simulink model "autopilot_simulink"  (R2016a)
settings: Solver=ode3  StartTime=0.0  StopTime=20  FixedStep=0.01  RelTol=1e-3
values from neighbouring files (symbols this model uses):
  Kx = KK(:,1:8)    [drone_config.m]
  Ky = KK(:,9:12)    [drone_config.m]
undefined symbols (not defined in the file or in its folder): sigbuilder_block
libraries: aerolibtransform2 x1, aerolib6dof2 x1
settings Model: Creator=rcasado  LastModifiedBy=rcasado
settings DataIOCC: LimitDataPoints=on  SaveFormat=Array
settings DebuggingCC: MultiTaskRateTransMsg=warning  AllowSymbolicDim=off
settings HardwareCC: ProdBitPerPointer=32  ProdLargestAtomicFloat=None  ProdIntDivRoundTo=Undefined  ProdEndianess=Unspecified  ProdWordSize=32  ProdHWDeviceType=32-bit Generic
settings ModelReferenceCC: PropagateSignalLabelsOutOfModel=off
settings ConfigComp: CovModelRefEnable=Off

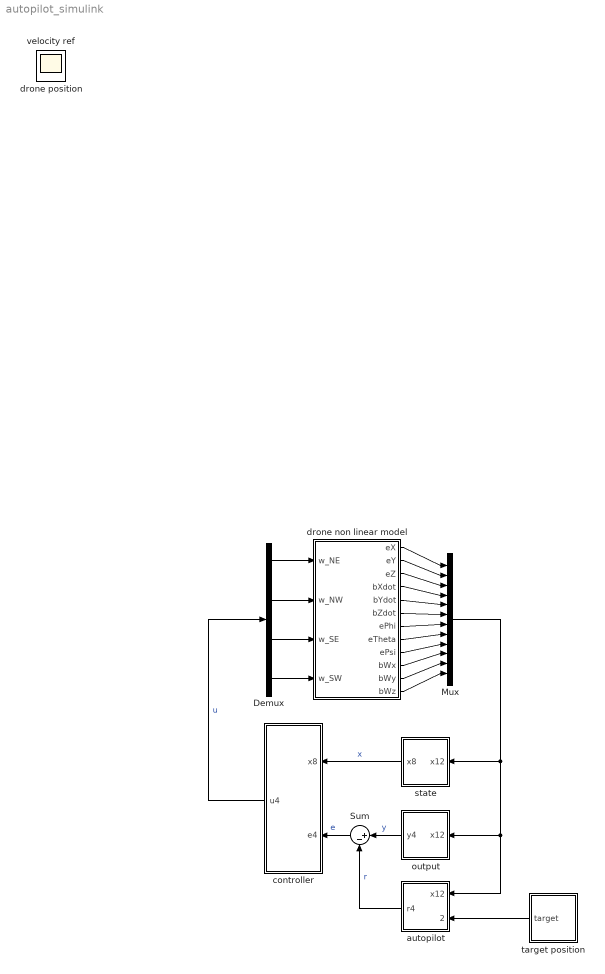
== system autopilot_simulink ==
  Demux : Demux
  Mux : Mux  Inputs=12
  Sum : Sum  Inputs=|+-
  autopilot : Subsystem
  controller : Subsystem
  drone non linear model : Subsystem
  output : Subsystem
  state : Subsystem
  target position : Subsystem
  drone position : Scope
  velocity ref : Scope
  wires:
  Mux/1 -> autopilot/1(x12), output/1(x12), state/1(x12)
  autopilot/1(r4) -> Sum/2  "r"
  output/1(y4) -> Sum/1  "y"
  state/1(x8) -> controller/1(x8)  "x"
  Sum/1 -> controller/2(e4)  "e"
  drone non linear model/1(eX) -> Mux/1
  drone non linear model/3(eZ) -> Mux/3
  drone non linear model/2(eY) -> Mux/2
  Demux/1 -> drone non linear model/1(w_NE)
  Demux/2 -> drone non linear model/2(w_NW)
  Demux/3 -> drone non linear model/3(w_SE)
  Demux/4 -> drone non linear model/4(w_SW)
  drone non linear model/12(bWz) -> Mux/12
  drone non linear model/11(bWy) -> Mux/11
  drone non linear model/4(bXdot) -> Mux/4
  drone non linear model/5(bYdot) -> Mux/5
  drone non linear model/6(bZdot) -> Mux/6
  drone non linear model/7(ePhi) -> Mux/7
  drone non linear model/8(eTheta) -> Mux/8
  drone non linear model/9(ePsi) -> Mux/9
  drone non linear model/10(bWx) -> Mux/10
  controller/1(u4) -> Demux/1  "u"
  target position/1(target) -> autopilot/2(target)

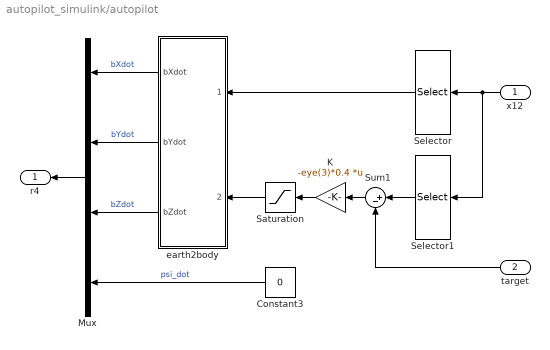
== system autopilot_simulink/autopilot ==
  x12 : Inport
  target : Inport  Port=2
  Constant3 : Constant  Value=0
  K : Gain  Gain=-eye(3)*0.4  Multiplication=Matrix(K*u)
  Mux : Mux
  Saturation : Saturate  UpperLimit=2  LowerLimit=-2
  Selector : Selector  InputPortWidth=12  IndexOptions=Index vector (dialog)  Indices=[7,8,9]  OutputSizes=1
  Selector1 : Selector  InputPortWidth=12  IndexOptions=Index vector (dialog)  Indices=[1;2;3]  OutputSizes=1
  Sum1 : Sum  Inputs=|+-
  earth2body : Subsystem
  r4 : Outport
  wires:
  Mux/1 -> r4/1
  Saturation/1 -> earth2body/2(eXYZdot)
  Constant3/1 -> Mux/4  "psi_dot"
  earth2body/2(bYdot) -> Mux/2  "bYdot"
  earth2body/1(bXdot) -> Mux/1  "bXdot"
  earth2body/3(bZdot) -> Mux/3  "bZdot"
  Selector1/1 -> Sum1/1
  K/1 -> Saturation/1
  Sum1/1 -> K/1
  x12/1 -> Selector1/1, Selector/1
  target/1 -> Sum1/2
  Selector/1 -> earth2body/1(orientation)

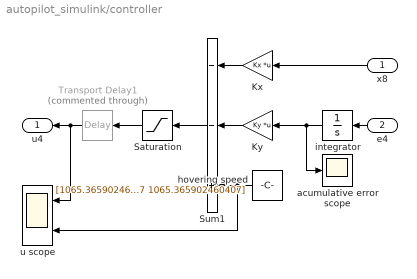
== system autopilot_simulink/controller ==
  x8 : Inport
  e4 : Inport  Port=2
  Kx : Gain  Gain=Kx  Multiplication=Matrix(K*u)
  Ky : Gain  Gain=Ky  Multiplication=Matrix(K*u)
  Saturation : Saturate  UpperLimit=1650  LowerLimit=0
  Sum1 : Sum  Inputs=--+
  Transport Delay1 : TransportDelay  Commented=through  DelayTime=0.05
  acumulative error scope : Scope
  hovering speed : Constant  Value=[1065.365902460407 1065.365902460407 1065.365902460407 1065.365902460407]
  integrator : Integrator
  u scope : Scope  NumInputPorts=2
  u4 : Outport
  wires:
  Saturation/1 -> Transport Delay1/1
  Kx/1 -> Sum1/1
  x8/1 -> Kx/1
  hovering speed/1 -> u scope/2, Sum1/3
  Sum1/1 -> Saturation/1
  Transport Delay1/1 -> u scope/1, u4/1
  e4/1 -> integrator/1
  Ky/1 -> Sum1/2
  integrator/1 -> Ky/1, acumulative error scope/1

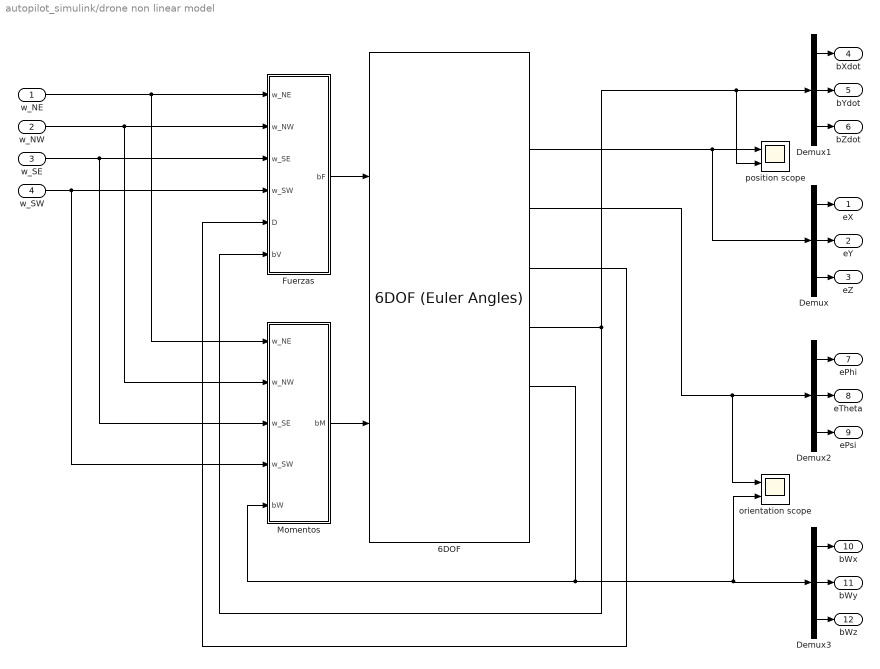
== system autopilot_simulink/drone non linear model ==
  w_NE : Inport
  w_NW : Inport  Port=2
  w_SE : Inport  Port=3
  w_SW : Inport  Port=4
  6DOF : aerolib6dof2/6DOF (Euler Angles)  units=Metric (MKS)  mtype=Fixed  rep=Euler Angles  xme_0=[0 0 10]  Vm_0=[0 0 0]  eul_0=[0 0 deg2rad(-30)]  pm_0=[0 0 0]  mass_0=1.840  mass_e=0.5  mass_f=2.0  inertia="[0.024916667  0  0 ; 0 0.024916667 0 ; 0 0 0.049066667]"  inertia_e=eye(3)  inertia_f=2*eye(3)  k_quat=1.0  vre_flag=on
  Demux{,1..3} (4 alike) : Demux  Outputs=3
  Fuerzas : Subsystem
  Momentos : Subsystem
  orientation scope : Scope  NumInputPorts=2
  position scope : Scope  NumInputPorts=2
  eX : Outport
  eY : Outport  Port=2
  eZ : Outport  Port=3
  bXdot : Outport  Port=4
  bYdot : Outport  Port=5
  bZdot : Outport  Port=6
  ePhi : Outport  Port=7
  eTheta : Outport  Port=8
  ePsi : Outport  Port=9
  bWx : Outport  Port=10
  bWy : Outport  Port=11
  bWz : Outport  Port=12
  wires:
  6DOF/2 -> Demux/1, position scope/1
  Momentos/1(bM) -> 6DOF/2
  w_NE/1 -> Momentos/1(w_NE), Fuerzas/1(w_NE)
  w_NW/1 -> Momentos/2(w_NW), Fuerzas/2(w_NW)
  w_SE/1 -> Momentos/3(w_SE), Fuerzas/3(w_SE)
  w_SW/1 -> Momentos/4(w_SW), Fuerzas/4(w_SW)
  6DOF/4 -> Fuerzas/5(D)
  Fuerzas/1(bF) -> 6DOF/1
  6DOF/6 -> Demux3/1, orientation scope/2, Momentos/5(bW)
  Demux/1 -> eX/1
  Demux/2 -> eY/1
  Demux/3 -> eZ/1
  6DOF/5 -> position scope/2, Demux1/1, Fuerzas/6(bV)
  Demux1/1 -> bXdot/1
  Demux1/2 -> bYdot/1
  Demux1/3 -> bZdot/1
  Demux2/1 -> ePhi/1
  Demux2/2 -> eTheta/1
  Demux2/3 -> ePsi/1
  Demux3/1 -> bWx/1
  Demux3/2 -> bWy/1
  Demux3/3 -> bWz/1
  6DOF/3 -> orientation scope/1, Demux2/1

== system autopilot_simulink/output ==
  x12 : Inport
  Selector : Selector  InputPortWidth=12  IndexOptions=Index vector (dialog)  Indices=[4 5 6 12]  OutputSizes=1
  y4 : Outport
  wires:
  x12/1 -> Selector/1
  Selector/1 -> y4/1

== system autopilot_simulink/state ==
  x12 : Inport
  Selector : Selector  InputPortWidth=12  IndexOptions=Index vector (dialog)  Indices=[7 8 10 11 12 4 5 6]  OutputSizes=1
  x8 : Outport
  wires:
  x12/1 -> Selector/1
  Selector/1 -> x8/1

== system autopilot_simulink/target position ==
  Mux1 : Mux  Inputs=3
  target position : Subsystem  Tag=STV Subsys  LoadFcn=sigbuilder_block('load',[514.2 0.6 340.2 585.6 ]);  StartFcn=sigbuilder_block('start');  StopFcn=sigbuilder_block('stop');  ClipboardFcn=sigbuilder_block('clipboard');  mask(Sigbuilder block){}
      mask help: Simulink:masks:SigbuilderBlock_MD
      mask init:
      | if ~strcmp(get_param(bdroot(gcbh),'SimulationStatus'),'stopped') tuvar = sigbuilder_block('maskInit'); end
      settings: CopyFcn=sigbuilder_block('copy');  DeleteFcn=sigbuilder_block('delete');  ModelCloseFcn=sigbuilder_block('modelClose');  PreSaveFcn=sigbuilder_block('preSave');  PauseFcn=sigbuilder_block('pause');  ContinueFcn=sigbuilder_block('continue');  NameChangeFcn=sigbuilder_block('namechange');  OpenFcn=sigbuilder_block('open',[514.2 0.6 375 585.6 ]);  CloseFcn=sigbuilder_block('close');
      mask Display: plot(0, 0, 100, 100,[2, 2, 32, 32, 2], [68, 8, 8, 68, 68],[32, 2], [38, 38], [32, 19, 2],[53, 60, 44], [32, 17, 17, 2],[16, 16, 31, 31]);txt = getActiveGroup(gcbh);text(2, 100, txt,'verticalAlignment', 'top');
  target : Outport
  wires:
  target position/3(pos_z) -> Mux1/3
  target position/1(pos_x) -> Mux1/1
  target position/2(pos_y) -> Mux1/2
  Mux1/1 -> target/1

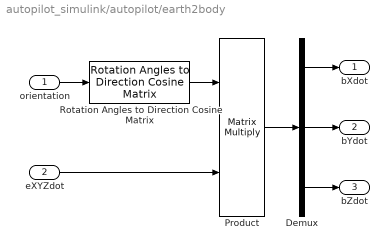
== system autopilot_simulink/autopilot/earth2body ==
  orientation : Inport
  eXYZdot : Inport  Port=2
  Demux : Demux  Outputs=3
  Product : Product  Multiplication=Matrix(*)
  Rotation Angles to Direction Cosine Matrix : aerolibtransform2/Rotation Angles to Direction Cosine Matrix  rotationOrder=XYZ
  bXdot : Outport
  bYdot : Outport  Port=2
  bZdot : Outport  Port=3
  wires:
  Product/1 -> Demux/1
  Rotation Angles to Direction Cosine Matrix/1 -> Product/1
  eXYZdot/1 -> Product/2
  orientation/1 -> Rotation Angles to Direction Cosine Matrix/1
  Demux/1 -> bXdot/1
  Demux/2 -> bYdot/1
  Demux/3 -> bZdot/1

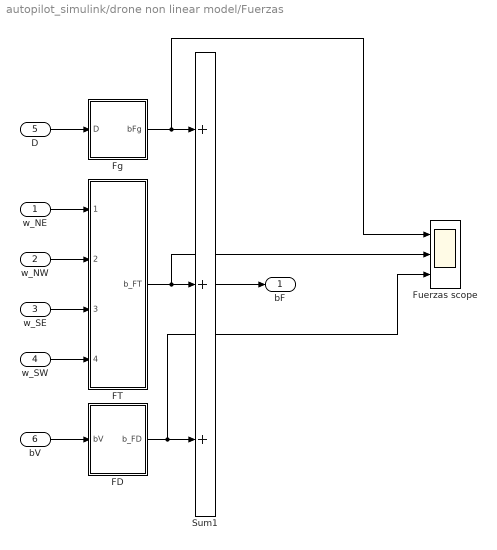
== system autopilot_simulink/drone non linear model/Fuerzas ==
  w_NE : Inport
  w_NW : Inport  Port=2
  w_SE : Inport  Port=3
  w_SW : Inport  Port=4
  D : Inport  Port=5
  bV : Inport  Port=6
  FD : Subsystem
  FT : Subsystem
  Fg : Subsystem
  Fuerzas scope : Scope  NumInputPorts=3
  Sum1 : Sum  Inputs=+++
  bF : Outport
  wires:
  D/1 -> Fg/1(D)
  Fg/1(bFg) -> Fuerzas scope/1, Sum1/1
  FT/1(b_FT) -> Fuerzas scope/2, Sum1/2
  w_SW/1 -> FT/4(w_SW)
  w_NE/1 -> FT/1(w_NE)
  w_SE/1 -> FT/3(w_SE)
  w_NW/1 -> FT/2(w_NW)
  Sum1/1 -> bF/1
  bV/1 -> FD/1(bV)
  FD/1(b_FD) -> Sum1/3, Fuerzas scope/3

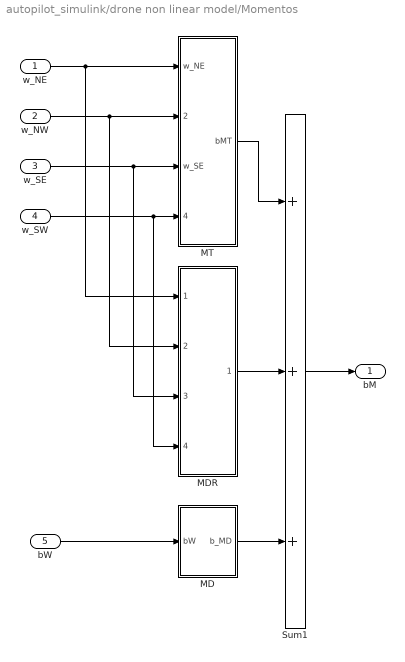
== system autopilot_simulink/drone non linear model/Momentos ==
  w_NE : Inport
  w_NW : Inport  Port=2
  w_SE : Inport  Port=3
  w_SW : Inport  Port=4
  bW : Inport  Port=5
  MD : Subsystem
  MDR : Subsystem
  MT : Subsystem
  Sum1 : Sum  Inputs=+++
  bM : Outport
  wires:
  bW/1 -> MD/1(bW)
  MT/1(bMT) -> Sum1/1
  w_SW/1 -> MDR/4(w_SW), MT/4(w_SW)
  w_NE/1 -> MDR/1(w_NE), MT/1(w_NE)
  w_SE/1 -> MDR/3(w_SE), MT/3(w_SE)
  w_NW/1 -> MDR/2(w_NW), MT/2(w_NW)
  Sum1/1 -> bM/1
  MD/1(b_MD) -> Sum1/3
  MDR/1(b_MDR) -> Sum1/2

== system autopilot_simulink/target position/target position ==
  Demux : Demux  Tag=STV Demux  Outputs=3
  FromWs : FromWorkspace  Tag=STV FromWs  VariableName=tuvar  SampleTime=0
      SigBuilderData=|
      | common.afterFinalStr = 'Extrapolate'
      | common.sampleTime = 0
      | dataSet(1).timeRange = [0 20]
      | dataSet(1).name = 've y aterriza'
      | dataSet(2).timeRange = [0 10]
      | dataSet(2).name = 'avanza1'
      | sbobj.Groups(1).Name = 've y aterriza'
      | sbobj.Groups(1).Signals(1).Name = 'pos_x'
      | sbobj.Groups(1).Signals(1).XData = [0 20]
      | sbobj.Groups(1).Signals(1).YData = [4 4]
      | sbobj.Groups(1).Signals(2).Name = 'pos_y'
      | sbobj.Groups(1).Signals(2).XData = [0 5 20]
      | sbobj.Groups(1).Signals(2).YData = [0 4 4]
      | sbobj.Groups(1).Signals(3).Name = 'pos_z'
      | sbobj.Groups(1).Signals(3).XData = [0 5 15 20]
      | sbobj.Groups(1).Signals(3).YData = [10 10 0 0]
      | sbobj.Groups(1).TimeRange = [0 20]
      | sbobj.Groups(2).Name = 'avanza1'
      | sbobj.Groups(2).Signals(1).Name = 'pos_x'
      | sbobj.Groups(2).Signals(1).XData = [0 1 1 4 6 10]
      | sbobj.Groups(2).Signals(1).YData = [0 0 3 3 3 3]
      | sbobj.Groups(2).Signals(2).Name = 'pos_y'
      | sbobj.Groups(2).Signals(2).XData = [0 4 10]
      | sbobj.Groups(2).Signals(2).YData = [0 4 4]
      | sbobj.Groups(2).Signals(3).Name = 'pos_z'
      | sbobj.Groups(2).Signals(3).XData = [0 6 6 10]
      | sbobj.Groups(2).Signals(3).YData = [10 10 0 0]
  pos_x : Outport  Tag=STV Outport
  pos_y : Outport  Tag=STV Outport  Port=2
  pos_z : Outport  Tag=STV Outport  Port=3
  wires:
  FromWs/1 -> Demux/1
  Demux/1 -> pos_x/1
  Demux/2 -> pos_y/1
  Demux/3 -> pos_z/1

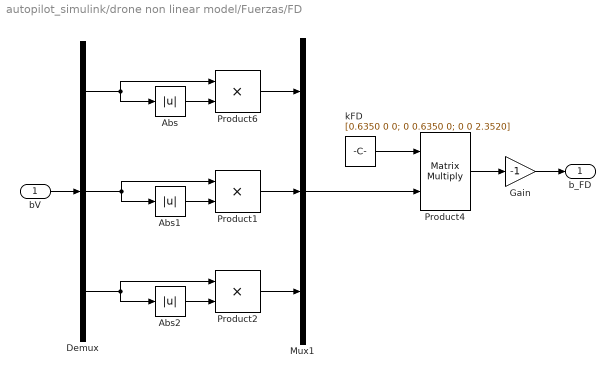
== system autopilot_simulink/drone non linear model/Fuerzas/FD ==
  bV : Inport
  Abs : Abs
  Abs1 : Abs
  Abs2 : Abs
  Demux : Demux  Outputs=3
  Gain : Gain  Gain=-1
  Mux1 : Mux  Inputs=3
  Product1 : Product
  Product2 : Product
  Product4 : Product  Multiplication=Matrix(*)
  Product6 : Product
  kFD : Constant  Value=[0.6350 0 0; 0 0.6350 0; 0 0 2.3520]
  b_FD : Outport
  wires:
  kFD/1 -> Product4/1
  Product4/1 -> Gain/1
  Mux1/1 -> Product4/2
  Product1/1 -> Mux1/2
  bV/1 -> Demux/1
  Abs/1 -> Product6/2
  Abs1/1 -> Product1/2
  Abs2/1 -> Product2/2
  Demux/1 -> Product6/1, Abs/1
  Demux/2 -> Product1/1, Abs1/1
  Demux/3 -> Product2/1, Abs2/1
  Product6/1 -> Mux1/1
  Product2/1 -> Mux1/3
  Gain/1 -> b_FD/1

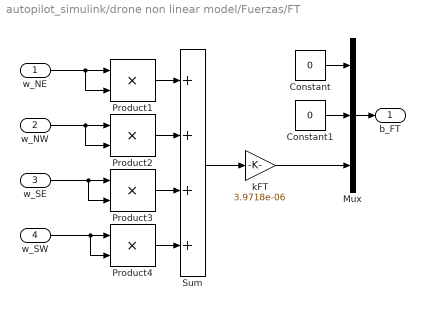
== system autopilot_simulink/drone non linear model/Fuerzas/FT ==
  w_NE : Inport
  w_NW : Inport  Port=2
  w_SE : Inport  Port=3
  w_SW : Inport  Port=4
  Constant : Constant  Value=0
  Constant1 : Constant  Value=0
  Mux : Mux  Inputs=3
  Product{1..4} (4 alike) : Product
  Sum : Sum  Inputs=++++
  kFT : Gain  Gain=3.9718e-06
  b_FT : Outport
  wires:
  Product4/1 -> Sum/4
  Product3/1 -> Sum/3
  Product2/1 -> Sum/2
  w_NW/1 -> Product2/2, Product2/1
  w_NE/1 -> Product1/2, Product1/1
  Product1/1 -> Sum/1
  Mux/1 -> b_FT/1
  w_SE/1 -> Product3/2, Product3/1
  w_SW/1 -> Product4/2, Product4/1
  Sum/1 -> kFT/1
  Constant/1 -> Mux/1
  Constant1/1 -> Mux/2
  kFT/1 -> Mux/3

== system autopilot_simulink/drone non linear model/Fuerzas/Fg ==
  D : Inport
  Fg scope : Scope  Commented=on  NumInputPorts=2
  Product : Product  Multiplication=Matrix(*)
  g : Gain  Gain=[0; 0; -9.8]
  masa : Constant  Value=1.840
  bFg : Outport
  wires:
  Product/1 -> Fg scope/2, bFg/1
  D/1 -> Product/1
  masa/1 -> g/1
  g/1 -> Fg scope/1, Product/2  "Fg"

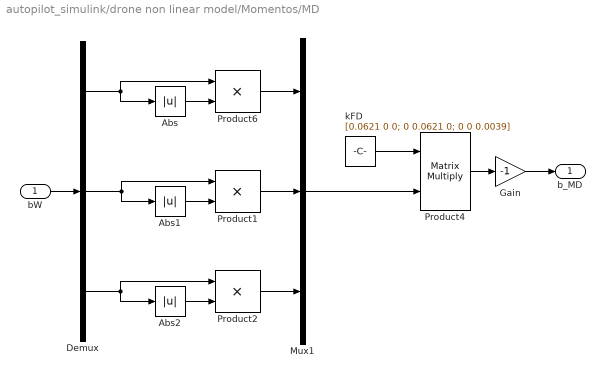
== system autopilot_simulink/drone non linear model/Momentos/MD ==
  bW : Inport
  Abs : Abs
  Abs1 : Abs
  Abs2 : Abs
  Demux : Demux  Outputs=3
  Gain : Gain  Gain=-1
  Mux1 : Mux  Inputs=3
  Product1 : Product
  Product2 : Product
  Product4 : Product  Multiplication=Matrix(*)
  Product6 : Product
  kFD : Constant  Value=[0.0621 0 0; 0 0.0621 0; 0 0 0.0039]
  b_MD : Outport
  wires:
  kFD/1 -> Product4/1
  Product4/1 -> Gain/1
  Mux1/1 -> Product4/2
  Product1/1 -> Mux1/2
  bW/1 -> Demux/1
  Abs/1 -> Product6/2
  Abs1/1 -> Product1/2
  Abs2/1 -> Product2/2
  Demux/1 -> Product6/1, Abs/1
  Demux/2 -> Product1/1, Abs1/1
  Demux/3 -> Product2/1, Abs2/1
  Product6/1 -> Mux1/1
  Product2/1 -> Mux1/3
  Gain/1 -> b_MD/1

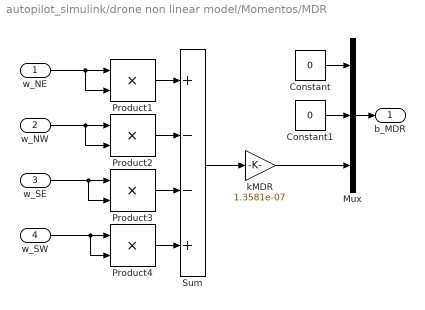
== system autopilot_simulink/drone non linear model/Momentos/MDR ==
  w_NE : Inport
  w_NW : Inport  Port=2
  w_SE : Inport  Port=3
  w_SW : Inport  Port=4
  Constant : Constant  Value=0
  Constant1 : Constant  Value=0
  Mux : Mux  Inputs=3
  Product{1..4} (4 alike) : Product
  Sum : Sum  Inputs=+--+
  kMDR : Gain  Gain=1.3581e-07
  b_MDR : Outport
  wires:
  Product4/1 -> Sum/4
  Product3/1 -> Sum/3
  Product2/1 -> Sum/2
  w_NW/1 -> Product2/2, Product2/1
  w_NE/1 -> Product1/2, Product1/1
  Product1/1 -> Sum/1
  Mux/1 -> b_MDR/1
  w_SE/1 -> Product3/2, Product3/1
  w_SW/1 -> Product4/2, Product4/1
  Sum/1 -> kMDR/1
  Constant/1 -> Mux/1
  Constant1/1 -> Mux/2
  kMDR/1 -> Mux/3

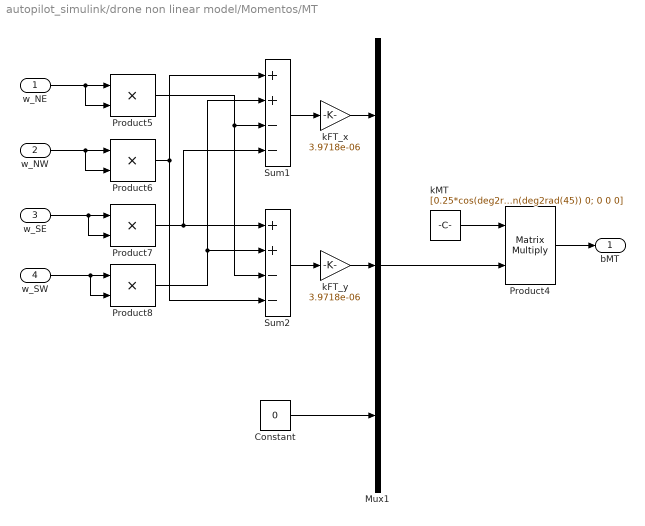
== system autopilot_simulink/drone non linear model/Momentos/MT ==
  w_NE : Inport
  w_NW : Inport  Port=2
  w_SE : Inport  Port=3
  w_SW : Inport  Port=4
  Constant : Constant  Value=0
  Mux1 : Mux  Inputs=3
  Product4 : Product  Multiplication=Matrix(*)
  Product{5..8} (4 alike) : Product
  Sum1 : Sum  Inputs=++--
  Sum2 : Sum  Inputs=++--
  kFT_x : Gain  Gain=3.9718e-06
  kFT_y : Gain  Gain=3.9718e-06
  kMT : Constant  Value=[0.25*cos(deg2rad(45)) 0 0; 0 0.25*sin(deg2rad(45)) 0; 0 0 0]
  bMT : Outport
  wires:
  kMT/1 -> Product4/1
  Product4/1 -> bMT/1
  Product8/1 -> Sum1/2, Sum2/2
  Product7/1 -> Sum2/1, Sum1/4
  w_NW/1 -> Product6/2, Product6/1
  w_NE/1 -> Product5/2, Product5/1
  Product6/1 -> Sum2/4, Sum1/1
  Mux1/1 -> Product4/2
  w_SE/1 -> Product7/2, Product7/1
  w_SW/1 -> Product8/2, Product8/1
  kFT_y/1 -> Mux1/2
  Sum1/1 -> kFT_x/1
  Sum2/1 -> kFT_y/1
  Product5/1 -> Sum2/3, Sum1/3
  kFT_x/1 -> Mux1/1
  Constant/1 -> Mux1/3
